simulink model "lab4_PID"  (Simulink 7.5)
settings: Solver=ode3  StartTime=0.0  StopTime=inf  FixedStep=.008  RelTol=1e-3
undefined symbols (not defined in the file): Serial_Port, Standard_Devices
libraries: rtwinlib x2, simulink x1
settings Model: Creator=Jenna Toennies  LastModifiedBy=Lou Kratchman  SimulationMode=external  ExtModeTrigDuration=1000000
settings DebuggingCC: StrictBusMsg=Warning
settings HardwareCC: ProdIntDivRoundTo=Zero  ProdEndianess=LittleEndian  ProdHWDeviceType=Generic->32-bit x86 compatible
settings RTWCC: SystemTargetFile=rtwin.tlc  TemplateMakefile=rtwin.tmf  Description=Real-Time Windows Target  ProcessScript=rtwin_make_rtw_hook  RTWCompilerOptimization=On
settings CodeAppCC: MaxIdLength=95
settings RTWinTargetCC: TargetLibSuffix=_rtwin.lib  TargetPreCompLibLocation=C:\Program Files\MATLAB\R2010a\toolbox\rtw\targets\rtwin\lib  TargetFunctionLibrary=ANSI_C  ERTCodeCoverageTool=None  PortableWordSizes=off

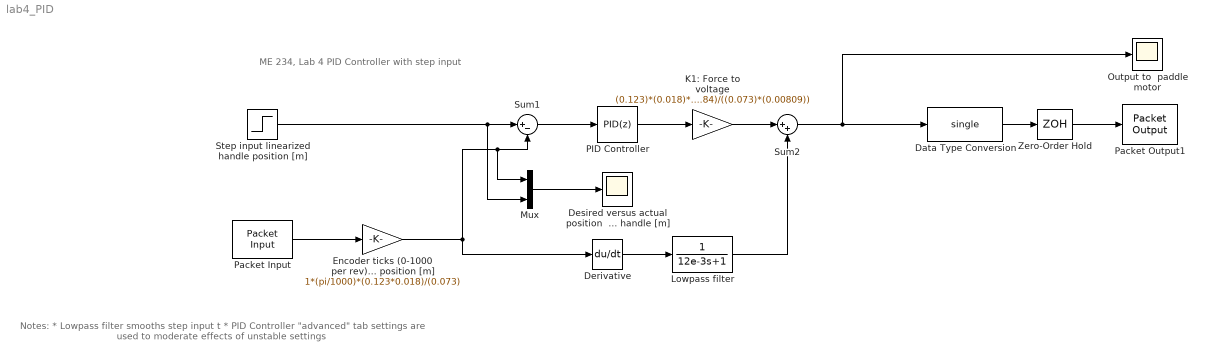
== system lab4_PID ==
  note: ME 234, Lab 4
      | PID Controller with step input
  note: Notes:
      | * Lowpass filter smooths step input t
      | * PID Controller "advanced" tab settings are used to moderate effects of unstable settings
  Data Type Conversion : DataTypeConversion  OutDataTypeMode=single  OutDataType=fixdt(1, 16)  OutScaling=2^0  OutDataTypeStr=single
  Derivative : Derivative
  Desired versus actual position  of paddle handle [m] : Scope
      settings: TimeRange=1  YMin=0.008  YMax=0.008018
  "Encoder ticks (0-1000 per rev)  to paddle position [m] " : Gain  Gain=1*(pi/1000)*(0.123*0.018)/(0.073)  ParameterDataType=fixdt(1, 16)  ParameterScaling=2^0  OutDataTypeMode=double  OutDataType=fixdt(1, 16)  OutScaling=2^0  OutDataTypeStr=double
  K1: Force to voltage : Gain  Gain=(0.123)*(0.018)*(1.84)/((0.073)*(0.00809))  ParameterDataType=fixdt(1, 16)  ParameterScaling=2^0  OutDataTypeMode=double  OutDataType=fixdt(1, 16)  OutScaling=2^0  OutDataTypeStr=double
  Lowpass filter : TransferFcn  Denominator=[12e-3 1]
  Mux : Mux  Inputs=2
  Output to  paddle motor : Scope
      settings: YMin=-1  YMax=3.75  SaveName=ScopeData2
  PID Controller : simulink/Continuous/PID Controller  DialogController=pidpack.PIDConfig.pidDDGCreate  DialogControllerArgs=DataTag0  SystemSampleTime=-1  Controller=PID  TimeDomain=Discrete-time  SampleTime=0.008  IntegratorMethod=Forward Euler  FilterMethod=Forward Euler  Form=Ideal  P=30  I=0  D=0.02  N=25  InitialConditionSource=internal  InitialConditionForIntegrator=0  InitialConditionForFilter=0  ExternalReset=none  LimitOutput=off  UpperSaturationLimit=2  LowerSaturationLimit=-2  LinearizeAsGain=off  AntiWindupMode=clamping  Kb=1  TrackingMode=off  Kt=1  PParamMin=[]  PParamMax=[]  IParamMin=[]  IParamMax=[]  DParamMin=[]  DParamMax=[]  NParamMin=[]  NParamMax=[]  KbParamMin=[]  KbParamMax=[]  KtParamMin=[]  KtParamMax=[]  POutMin=[]  POutMax=[]  IOutMin=[]  IOutMax=[]  DOutMin=[]  DOutMax=[]  NOutMin=[]  NOutMax=[]  KbOutMin=[]  KbOutMax=[]  KtOutMin=[]  KtOutMax=[]  IntegratorOutMin=[]  IntegratorOutMax=[]  FilterOutMin=[]  FilterOutMax=[]  SumOutMin=[]  SumOutMax=[]  SumI1OutMin=[]  SumI1OutMax=[]  SumI2OutMin=[]  SumI2OutMax=[]  SumI3OutMin=[]  SumI3OutMax=[]  SumDOutMin=[]  SumDOutMax=[]  SaturationOutMin=[]  SaturationOutMax=[]  IntegratorContinuousStateAttributes=''  IntegratorStateMustResolveToSignalObject=off  IntegratorRTWStateStorageClass=Auto  FilterContinuousStateAttributes=''  FilterStateMustResolveToSignalObject=off  FilterRTWStateStorageClass=Auto
  Packet Input : rtwinlib/Packet Input  SampleTime=.008  DrvName=Standard_Devices/Serial_Port  DrvAddress=9  DrvOptions=[115200 8 0 0 0 0 0]  PacketSize=4  DataTypes='1*int32'  ShowReady=off  ShowError=off  PacketID=1  ShowTimestamp=off
      settings: AttributesFormatString=Standard Devices\nSerial Port [9h]
  Packet Output1 : rtwinlib/Packet Output  SampleTime=.008  DrvName=Standard_Devices/Serial_Port  DrvAddress=9  DrvOptions=[115200 8 0 0 0 0 0]  PacketSize=4  DataTypes='1*single'  ShowReady=off  ShowError=off  PacketID=1  InitialValue=[]  FinalValue=[]
      settings: AttributesFormatString=Standard Devices\nSerial Port [9h]
  Step input linearized handle position [m] : Step  Time=2  After=0.05  SampleTime=0.008
  Sum1 : Sum  Inputs=|+-  OutDataType=fixdt(1, 16)  OutScaling=2^0
  Sum2 : Sum  Inputs=|++  OutDataType=fixdt(1, 16)  OutScaling=2^0
  Zero-Order Hold : ZeroOrderHold  SampleTime=.008
  wires:
  Packet Input/1 -> "Encoder ticks (0-1000 per rev)  to paddle position [m] "/1
  Data Type Conversion/1 -> Zero-Order Hold/1
  Zero-Order Hold/1 -> Packet Output1/1
  "Encoder ticks (0-1000 per rev)  to paddle position [m] "/1 -> Sum1/2, Mux/1, Derivative/1
  Mux/1 -> Desired versus actual position  of paddle handle [m]/1
  Step input linearized handle position [m]/1 -> Sum1/1, Mux/2
  Sum1/1 -> PID Controller/1
  PID Controller/1 -> K1: Force to voltage/1
  Sum2/1 -> Data Type Conversion/1, Output to  paddle motor/1
  K1: Force to voltage/1 -> Sum2/1
  Derivative/1 -> Lowpass filter/1
  Lowpass filter/1 -> Sum2/2
